simulink model "LIM"  (R2022b)
settings: Solver=VariableStepAuto  StartTime=0.0  StopTime=2  RelTol=1e-3
model workspace (MAT data in the model file):
  F = Simulink.Parameter
  F.DataType = 'auto'
  F.Complexity = 'real'
  F.Dimensions = [0 0]
values from neighbouring files (symbols this model uses):
  B = 0.93    [proj.m]
  D = 2.150    (= 2.15)    [proj.m]
  Llr = 0.0323    [proj.m]
  Lls = 0.0788    [proj.m]
  Lm = 0.0420    (= 0.042)    [proj.m]
  M = 16.1    [proj.m]
  P = 2    [proj.m]
  Rr = 10.166    [proj.m]
  Rs = 1.6875    [proj.m]
  Vo = 220    [proj.m]
  Ws = 314.5    [proj.m]
libraries: spspowerguiLib x1
settings Model: Creator=Hassan Alam  LastModifiedBy=DELL
settings SolverCC: AlgebraicLoopSolver=TrustRegion
settings DebuggingCC: UnconnectedInputMsg=warning  UnconnectedOutputMsg=warning  UnconnectedLineMsg=warning  SFMachineParentedDataDiag=warning  ArithmeticOperatorsInVariantConditions=warning
settings ModelReferenceCC: EnableRefExpFcnMdlSchedulingChecks=on
settings SFSimCC: CustomCodeUndefinedFunction=UseInterfaceOnly
settings RTWCC: DLArmComputeVersion=19.05

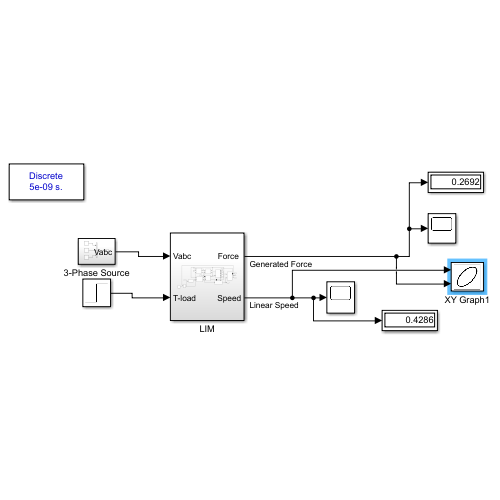
[thumbnail: Simulink's stored preview of the top-level diagram]
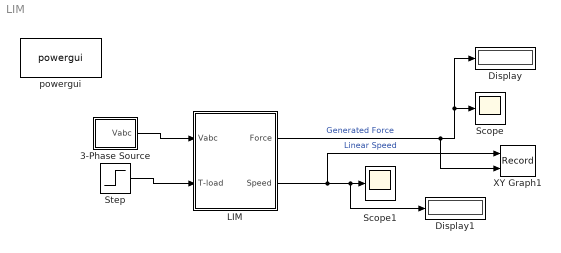
== system LIM ==
  3-Phase Source : Subsystem
  Display : Display
  Display1 : Display
  LIM : Subsystem
  Scope : Scope
  Scope1 : Scope
  Step : Step  Time=2  After=2  SampleTime=0
  XY Graph1 : Record  FileSettingsInternal="{\"entries\":[{\"content\":{\"excelSettings\":{\"content\":{},\"type\":\"Streamout.ExcelSettings\"}},\"type\":\"Streamout.FileSettingStorage\",\"uuid\":\"f2251dd7-1574-4eda-90b9-688bc1165eb5\"}],\"packageUris\":[\"http://schema.mathworks.com/mf0/streamout_blocks/R2020a\"],\"version\":\"1.0\"}"  Layout=[1 1]  SignalsInternal="{\"entries\":[{\"content\":{\"signals\":[{\"content\":{\"blockPath\":[\"Linear_IM/XY Graph1\"],\"channel\":[],\"dimensions\":[1],\"domain\":\"Linear_IM/XY Graph1\",\"lineColor\":\"#a2142f\",\"plots\":[1],\"port\":1,\"sid\":[],\"signalID\":8,\"signalName\":\"Linear Speed\"},\"type\":\"RecordBlkView.Signal\",\"uuid\":\"07500a95-6970-4b1d-b2d0-133414292f8e\"},{\"content\":{\"blockPath\":[\"Linear_IM/XY Graph1\"],\"channel\":[],\"dimensions\":[1],\"domain\":\"Linear_IM/XY Graph1\",\"lineColor\":\"#139fff\",\"plots\":[1],\"port\":2,\"sid\":[],\"signalID\":11,\"signalName\":\"Generated Force\"},\"type\":\"RecordBlkView.Signal\",\"uuid\":\"d5d04c6d-1390-4e30-b79d-0de345d9fcfb\"}]},\"type\":\"RecordBlkView.InputSignals\",\"uuid\":\"6577f966-2e08-44dc-8997-1caec95d4b14\"}],\"packageUris\":[\"http://schema.mathworks.com/mf0/streamout_blocks/R2020a\"],\"version\":\"1.0\"}"  VisualizationBindings="{\"xyplotplugin\":{\"info\":[{\"series\":[{\"bindingParametersList\":[{\"parameter\":\"X-Axis\",\"signalID\":8,\"signalName\":\"Linear Speed\"},{\"parameter\":\"Y-Axis\",\"signalID\":11,\"signalName\":\"Generated Force\"}],\"seriesID\":8522}],\"subplotID\":1}]}}"  CompatibilityTag=XY
  powergui : spspowerguiLib/powergui  Priority=1  SimulationMode=Discrete  SampleTime=50e-10  frequency=60  Iterations=50  frequencyindice=60  Pbase=100e6  ErrMax=1e-4  UnitsV=kV  UnitsW=MW  buscounter=0  FunctionMessages=off  echomessages=off  EnableUseOfTLC=off  CurrentSourceSwitches=off  DisableSnubberDevices=off  DisableRonSwitches=off  DisableVfSwitches=off  DisplayEquations=off  AutomaticDiscreteSolvers=off  SolverType=Tustin/Backward Euler (TBE)  Interpol=off  ExternalGateDelay=off  methode=off  Ts=100  x0status=blocks  SPID=on  SwTol=0  HookPort=off  NonlinearTolerance=1e-4  nMaxIteration=100  ContinueOnMaxIteration=off  RestoreLinks=warning  ResistiveCurrentMeasurement=off  Frange=[0:2:500]  Ylog=off  Xlog=on  ShowGrid=off  save=off  variable=ZData  structure=0  ZoomFFT=off  StartTime=0.0  cycles=1  DisplayStyle=1  fundamental=60  FreqAxis=off  MaxFrequency=1000  frequencyindicesteady=1  RmsSteady=1  display=off
  wires:
  Step/1 -> LIM/2(T-load)
  LIM/1("Force ") -> XY Graph1/2, Display/1, Scope/1  "Generated Force"
  LIM/2(" Speed") -> XY Graph1/1, Scope1/1, Display1/1  "Linear Speed"
  3-Phase Source/1(Vabc) -> LIM/1(Vabc)

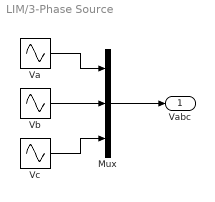
== system LIM/3-Phase Source ==
  Mux : Mux  Inputs=3
  Va : Sin  Amplitude=Vo  Frequency=Ws  SampleTime=0
  Vb : Sin  Amplitude=Vo  Frequency=Ws  Phase=-2*pi/3  SampleTime=0
  Vc : Sin  Amplitude=Vo  Frequency=Ws  Phase=2*pi/3  SampleTime=0
  Vabc : Outport
  wires:
  Mux/1 -> Vabc/1
  Vb/1 -> Mux/2
  Va/1 -> Mux/1
  Vc/1 -> Mux/3

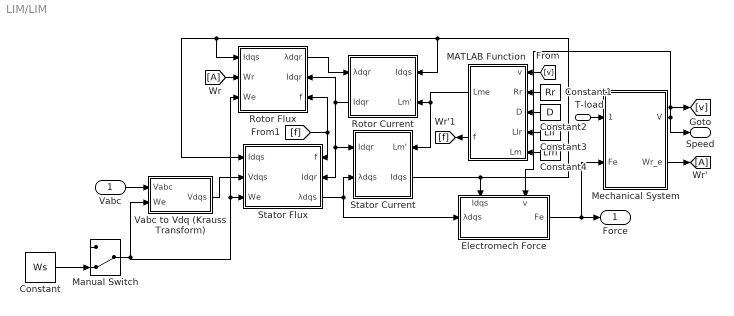
== system LIM/LIM ==
  Vabc : Inport
  T-load : Inport  Port=2
  Constant : Constant  Value=Ws
  Constant1 : Constant  Value=Rr
  Constant2 : Constant  Value=D
  Constant3 : Constant  Value=Llr
  Constant4 : Constant  Value=Lm
  Electromech Force : Subsystem
      settings: PortSchema="{\"entries\":[{\"content\":{\"sides\":[{\"content\":{\"connectorIds\":[\"In1\"]},\"type\":\"ConnectorPlacement.EquallySpacedRectSide\",\"uuid\":\"a4b29cca-9cb0-4324-9244-2049ffc93668\"},{\"content\":{\"connectorIds\":[\"Out1\"],\"side\":\"RIGHT\"},\"type\":\"ConnectorPlacement.EquallySpacedRectSide\",\"uuid\":\"b20ff3ac-d40e-4f59-bb91-f6f2c0c6ca63\"},{\"content\":{\"connectorIds\":[\"In2\",\"In3\"],\"side\":\"TOP\"},\"type\":\"ConnectorPlacement.EquallySpacedRectSide\",\"uuid\":\"55342d43-b8f9-4aa9-846c-26670e92f4ca\"},{\"content\":{\"connectorIds\":[],\"side\":\"HIDDEN\"},\"type\":\"ConnectorPlacement.EquallySpacedRectSide\",\"uuid\":\"5fed22a0-a45a-430c-a997-0be85a9315bb\"}]},\"type\":\"ConnectorPlacement.EquallySpacedConnector\",\"uuid\":\"78d5652d-2b6b-4c50-974b-d09ad892483f\"}],\"packageUris\":[\"http://schema.mathworks.com/mf0/Connector/R2020b\"],\"version\":\"1.0\"}"
  MATLAB Function : MATLAB Function  TreatAsAtomicUnit=on
  Manual Switch : ManualSwitch  CurrentSetting=0
  Mechanical System : Subsystem
  Rotor Current : Subsystem
      settings: PortSchema="{\"entries\":[{\"content\":{\"sides\":[{\"content\":{\"connectorIds\":[\"In1\",\"Out1\"]},\"type\":\"ConnectorPlacement.EquallySpacedRectSide\",\"uuid\":\"b9a9f404-9b3b-4182-a50e-1bf7cef191e8\"},{\"content\":{\"connectorIds\":[\"In2\",\"In3\"],\"side\":\"RIGHT\"},\"type\":\"ConnectorPlacement.EquallySpacedRectSide\",\"uuid\":\"68159d79-7975-4fd0-98a3-7e35432781a2\"},{\"content\":{\"connectorIds\":[],\"side\":\"TOP\"},\"type\":\"ConnectorPlacement.EquallySpacedRectSide\",\"uuid\":\"0c4dbb5d-b4d4-4876-b829-49090bd6eeb8\"},{\"content\":{\"connectorIds\":[],\"side\":\"BOTTOM\"},\"type\":\"ConnectorPlacement.EquallySpacedRectSide\",\"uuid\":\"e42509db-2e5f-42f8-9a91-9046ba95e836\"},{\"content\":{\"connectorIds\":[],\"side\":\"HIDDEN\"},\"type\":\"ConnectorPlacement.EquallySpacedRectSide\",\"uuid\":\"f2a65973-682a-4dd6-b429-3fa72198cae4\"}]},\"type\":\"ConnectorPlacement.EquallySpacedConnector\",\"uuid\":\"744eb17f-cf6a-4151-90db-78263b57d619\"}],\"packageUris\":[\"http://schema.mathworks.com/mf0/Connector/R2020b\"],\"version\":\"1.0\"}"
  Rotor Flux : Subsystem
      settings: PortSchema="{\"entries\":[{\"content\":{\"sides\":[{\"content\":{\"connectorIds\":[\"In1\",\"In2\",\"In3\"]},\"type\":\"ConnectorPlacement.EquallySpacedRectSide\",\"uuid\":\"b9a9f404-9b3b-4182-a50e-1bf7cef191e8\"},{\"content\":{\"connectorIds\":[\"Out1\",\"In4\",\"In5\"],\"side\":\"RIGHT\"},\"type\":\"ConnectorPlacement.EquallySpacedRectSide\",\"uuid\":\"68159d79-7975-4fd0-98a3-7e35432781a2\"},{\"content\":{\"connectorIds\":[],\"side\":\"TOP\"},\"type\":\"ConnectorPlacement.EquallySpacedRectSide\",\"uuid\":\"0c4dbb5d-b4d4-4876-b829-49090bd6eeb8\"},{\"content\":{\"connectorIds\":[],\"side\":\"HIDDEN\"},\"type\":\"ConnectorPlacement.EquallySpacedRectSide\",\"uuid\":\"f2a65973-682a-4dd6-b429-3fa72198cae4\"}]},\"type\":\"ConnectorPlacement.EquallySpacedConnector\",\"uuid\":\"744eb17f-cf6a-4151-90db-78263b57d619\"}],\"packageUris\":[\"http://schema.mathworks.com/mf0/Connector/R2020b\"],\"version\":\"1.0\"}"
  Stator Current : Subsystem
      settings: PortSchema="{\"entries\":[{\"content\":{\"sides\":[{\"content\":{\"connectorIds\":[\"In1\",\"In2\"]},\"type\":\"ConnectorPlacement.EquallySpacedRectSide\",\"uuid\":\"c6a8d684-b7d2-4173-9e8a-0a77b360fa3b\"},{\"content\":{\"connectorIds\":[\"In3\",\"Out1\"],\"side\":\"RIGHT\"},\"type\":\"ConnectorPlacement.EquallySpacedRectSide\",\"uuid\":\"6b547613-238c-47a7-9a25-113e0bcf67e8\"},{\"content\":{\"connectorIds\":[],\"side\":\"TOP\"},\"type\":\"ConnectorPlacement.EquallySpacedRectSide\",\"uuid\":\"9eb731ca-d22d-4bff-90d4-9f452150afc4\"},{\"content\":{\"connectorIds\":[],\"side\":\"HIDDEN\"},\"type\":\"ConnectorPlacement.EquallySpacedRectSide\",\"uuid\":\"3386087c-4273-46bf-b0bc-9959c9fde15b\"}]},\"type\":\"ConnectorPlacement.EquallySpacedConnector\",\"uuid\":\"3fded039-aa6e-4722-8a98-01f4cd5eabc0\"}],\"packageUris\":[\"http://schema.mathworks.com/mf0/Connector/R2020b\"],\"version\":\"1.0\"}"
  Stator Flux : Subsystem
      settings: PortSchema="{\"entries\":[{\"content\":{\"sides\":[{\"content\":{\"connectorIds\":[\"In1\",\"In2\",\"In3\"]},\"type\":\"ConnectorPlacement.EquallySpacedRectSide\",\"uuid\":\"a4b29cca-9cb0-4324-9244-2049ffc93668\"},{\"content\":{\"connectorIds\":[\"In4\",\"In5\",\"Out1\"],\"side\":\"RIGHT\"},\"type\":\"ConnectorPlacement.EquallySpacedRectSide\",\"uuid\":\"b20ff3ac-d40e-4f59-bb91-f6f2c0c6ca63\"},{\"content\":{\"connectorIds\":[],\"side\":\"TOP\"},\"type\":\"ConnectorPlacement.EquallySpacedRectSide\",\"uuid\":\"55342d43-b8f9-4aa9-846c-26670e92f4ca\"},{\"content\":{\"connectorIds\":[],\"side\":\"HIDDEN\"},\"type\":\"ConnectorPlacement.EquallySpacedRectSide\",\"uuid\":\"5fed22a0-a45a-430c-a997-0be85a9315bb\"}]},\"type\":\"ConnectorPlacement.EquallySpacedConnector\",\"uuid\":\"78d5652d-2b6b-4c50-974b-d09ad892483f\"}],\"packageUris\":[\"http://schema.mathworks.com/mf0/Connector/R2020b\"],\"version\":\"1.0\"}"
  Vabc to Vdq (Krauss Transform) : Subsystem
  Wr : From
  Wr' : Goto
  "Force " : Outport
  " Speed" : Outport  Port=2
  wires:
  Electromech Force/1(Fe) -> Mechanical System/2(Fe), "Force "/1
  T-load/1 -> Mechanical System/1(F-load)
  Mechanical System/1(V) -> Electromech Force/3(v), [v], " Speed"/1
  Stator Flux/1(λdqs) -> Stator Current/2(λdqs), Electromech Force/1(λdqs)
  Stator Current/1(Idqs) -> Rotor Flux/1(Idqs), Stator Flux/1(Idqs), Rotor Current/2(Idqs), Electromech Force/2(Idqs)
  Rotor Flux/1(λdqr) -> Rotor Current/1(λdqr)
  Rotor Current/1(Idqr) -> Rotor Flux/4(Idqr), Stator Flux/5(Idqr), Stator Current/1(Idqr)
  Wr/1 -> Rotor Flux/2(Wr)
  Vabc/1 -> Vabc to Vdq (Krauss Transform)/1(Vabc)
  Vabc to Vdq (Krauss Transform)/1(Vdqs) -> Stator Flux/2(Vdqs)
  MATLAB Function/1(Lme) -> Stator Current/3(Lm'), Rotor Current/3(Lm')
  [v] -> MATLAB Function/1(v)
  Constant1/1 -> MATLAB Function/2(Rr)
  Constant2/1 -> MATLAB Function/3(D)
  Constant3/1 -> MATLAB Function/4(Llr)
  Constant4/1 -> MATLAB Function/5(Lm)
  MATLAB Function/2(f) -> [f]
  [f] -> Rotor Flux/5(f), Stator Flux/4(f)
  Mechanical System/2(Wr_e) -> Wr'/1
  Manual Switch/1 -> Rotor Flux/3(We), Stator Flux/3(We), Vabc to Vdq (Krauss Transform)/2(We)
  Constant/1 -> Manual Switch/2

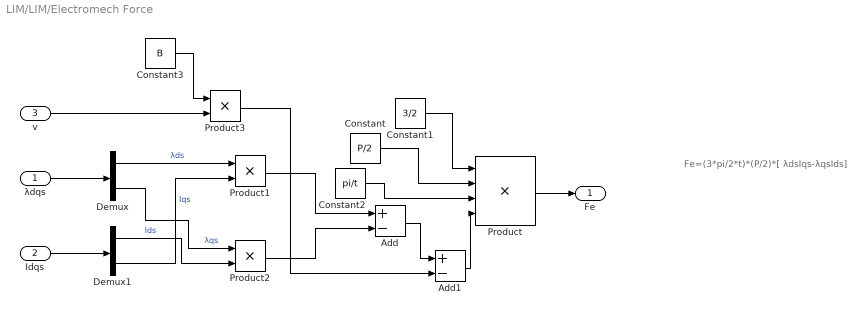
== system LIM/LIM/Electromech Force ==
  note: Fe=(3*pi/2*t)*(P/2)*[ λdsIqs-λqsIds]
  λdqs : Inport
  Idqs : Inport  Port=2
  v : Inport  Port=3
  Add : Sum  Inputs=+-
  Add1 : Sum  Inputs=+-
  Constant : Constant  Value=P/2
  Constant1 : Constant  Value=3/2
  Constant2 : Constant  Value=pi/t
  Constant3 : Constant  Value=B
  Demux : Demux  Outputs=2
  Demux1 : Demux  Outputs=2
  Product : Product  Inputs=4
  Product1 : Product
  Product2 : Product
  Product3 : Product
  Fe : Outport
  wires:
  Product/1 -> Fe/1
  Constant1/1 -> Product/1
  λdqs/1 -> Demux/1
  Idqs/1 -> Demux1/1
  Demux/1 -> Product1/1  "λds"
  Demux1/2 -> Product1/2  "Iqs"
  Demux/2 -> Product2/1  "λqs"
  Demux1/1 -> Product2/2  "Ids"
  Product1/1 -> Add/1
  Product2/1 -> Add/2
  Constant2/1 -> Product/3
  Constant/1 -> Product/2
  v/1 -> Product3/2
  Add/1 -> Add1/1
  Add1/1 -> Product/4
  Product3/1 -> Add1/2
  Constant3/1 -> Product3/1

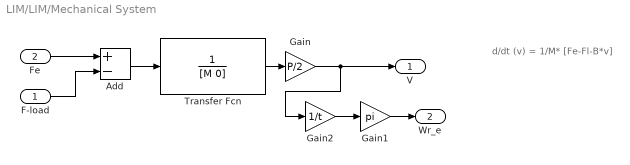
== system LIM/LIM/Mechanical System ==
  note: d/dt (v) = 1/M* [Fe-Fl-B*v]
  F-load : Inport
  Fe : Inport  Port=2
  Add : Sum  Inputs=+-
  Gain : Gain  Gain=P/2
  Gain1 : Gain  Gain=pi
  Gain2 : Gain  Gain=1/t
  Transfer Fcn : TransferFcn  Denominator=[M 0]
  V : Outport
  Wr_e : Outport  Port=2
  wires:
  Fe/1 -> Add/1
  F-load/1 -> Add/2
  Add/1 -> Transfer Fcn/1
  Gain2/1 -> Gain1/1
  Gain1/1 -> Wr_e/1
  Gain/1 -> Gain2/1, V/1
  Transfer Fcn/1 -> Gain/1

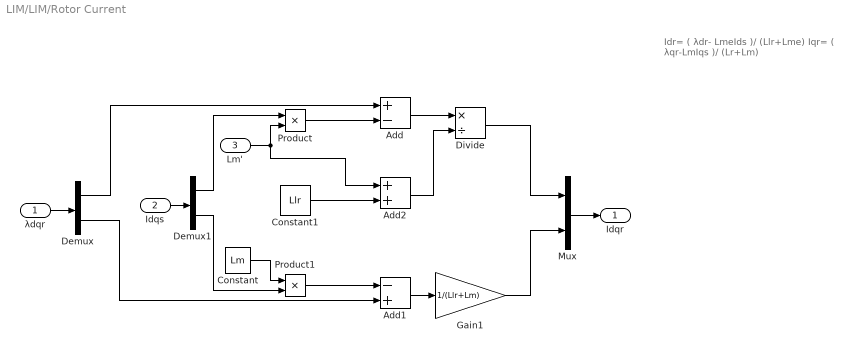
== system LIM/LIM/Rotor Current ==
  note: Idr= ( λdr- LmeIds )/ (Llr+Lme)
      |
      | Iqr= ( λqr-LmIqs )/ (Lr+Lm)
  λdqr : Inport
  Idqs : Inport  Port=2
  Lm' : Inport  Port=3
  Add : Sum  Inputs=+-
  Add1 : Sum  Inputs=-+
  Add2 : Sum
  Constant : Constant  Value=Lm  VectorParams1D=off
  Constant1 : Constant  Value=Llr
  Demux : Demux  Outputs=2
  Demux1 : Demux  Outputs=2
  Divide : Product  Inputs=*/
  Gain1 : Gain  Gain=1/(Llr+Lm)
  Mux : Mux  Inputs=2
  Product : Product
  Product1 : Product
  Idqr : Outport
  wires:
  Mux/1 -> Idqr/1
  λdqr/1 -> Demux/1
  Idqs/1 -> Demux1/1
  Demux1/1 -> Product/1
  Demux1/2 -> Product1/2
  Demux/1 -> Add/1
  Demux/2 -> Add1/2
  Product/1 -> Add/2
  Product1/1 -> Add1/1
  Add/1 -> Divide/1
  Add1/1 -> Gain1/1
  Gain1/1 -> Mux/2
  Divide/1 -> Mux/1
  Constant/1 -> Product1/1
  Constant1/1 -> Add2/2
  Lm'/1 -> Add2/1, Product/2
  Add2/1 -> Divide/2

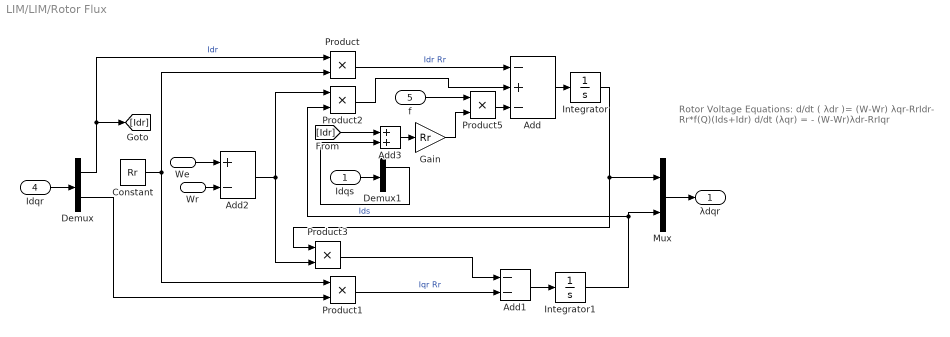
== system LIM/LIM/Rotor Flux ==
  note: Rotor Voltage Equations:
      | d/dt ( λdr )= (W-Wr) λqr-RrIdr- Rr*f(Q)(Ids+Idr)
      | d/dt (λqr) = - (W-Wr)λdr-RrIqr
  Idqs : Inport
  Wr : Inport  Port=2
  We : Inport  Port=3
  Idqr : Inport  Port=4
  f : Inport  Port=5
  Add : Sum  Inputs=-+-
  Add1 : Sum  Inputs=--
  Add2 : Sum  Inputs=+-
  Add3 : Sum
  Constant : Constant  Value=Rr
  Demux : Demux  Outputs=2
  Demux1 : Demux  Outputs=2
  Gain : Gain  Gain=Rr
  Integrator : Integrator
  Integrator1 : Integrator
  Mux : Mux  Inputs=2
  Product{,1..3,5} (5 alike) : Product
  λdqr : Outport
  wires:
  Mux/1 -> λdqr/1
  Idqr/1 -> Demux/1
  Demux/1 -> [Idr], Product/1  "Idr"
  Demux/2 -> Product1/2
  Constant/1 -> Product1/1, Product/2
  Product/1 -> Add/1  "Idr Rr"
  Product1/1 -> Add1/2  "Iqr Rr"
  Add/1 -> Integrator/1
  Add1/1 -> Integrator1/1
  Integrator1/1 -> Mux/2, Product2/2
  Integrator/1 -> Product3/1, Mux/1
  We/1 -> Add2/1
  Wr/1 -> Add2/2
  Add2/1 -> Product3/2, Product2/1
  Product2/1 -> Add/2
  Product3/1 -> Add1/1
  Demux1/1 -> Add3/2  "Ids"
  Product5/1 -> Add/3
  Add3/1 -> Gain/1
  Gain/1 -> Product5/2
  f/1 -> Product5/1
  Idqs/1 -> Demux1/1
  [Idr] -> Add3/1

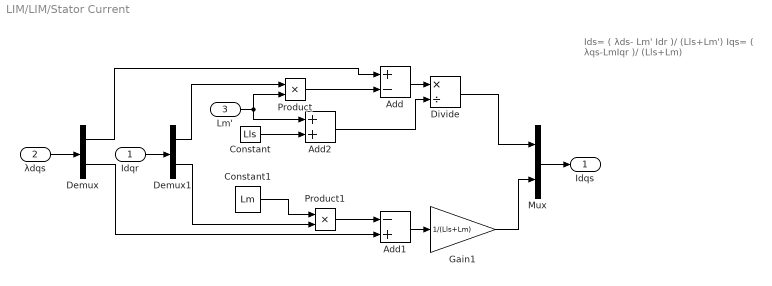
== system LIM/LIM/Stator Current ==
  note: Ids= ( λds- Lm' Idr )/ (Lls+Lm')
      |
      | Iqs= ( λqs-LmIqr )/ (Lls+Lm)
  Idqr : Inport
  λdqs : Inport  Port=2
  Lm' : Inport  Port=3
  Add : Sum  Inputs=+-
  Add1 : Sum  Inputs=-+
  Add2 : Sum
  Constant : Constant  Value=Lls
  Constant1 : Constant  Value=Lm  VectorParams1D=off
  Demux : Demux  Outputs=2
  Demux1 : Demux  Outputs=2
  Divide : Product  Inputs=*/
  Gain1 : Gain  Gain=1/(Lls+Lm)
  Mux : Mux  Inputs=2
  Product : Product
  Product1 : Product
  Idqs : Outport
  wires:
  Demux/2 -> Add1/2
  Demux1/1 -> Product/1
  Product/1 -> Add/2
  Product1/1 -> Add1/1
  λdqs/1 -> Demux/1
  Add1/1 -> Gain1/1
  Mux/1 -> Idqs/1
  Idqr/1 -> Demux1/1
  Demux/1 -> Add/1
  Demux1/2 -> Product1/2
  Add/1 -> Divide/1
  Divide/1 -> Mux/1
  Gain1/1 -> Mux/2
  Constant1/1 -> Product1/1
  Lm'/1 -> Add2/1, Product/2
  Constant/1 -> Add2/2
  Add2/1 -> Divide/2

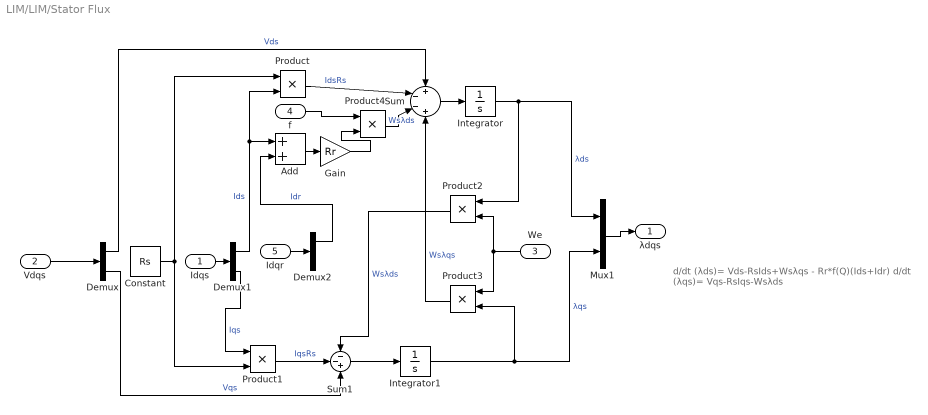
== system LIM/LIM/Stator Flux ==
  note: d/dt (λds)= Vds-RsIds+Wsλqs - Rr*f(Q)(Ids+Idr)
      |
      | d/dt (λqs)= Vqs-RsIqs-Wsλds
  Idqs : Inport
  Vdqs : Inport  Port=2
  We : Inport  Port=3
  f : Inport  Port=4
  Idqr : Inport  Port=5
  Add : Sum
  Constant : Constant  Value=Rs
  Demux : Demux  Outputs=2
  Demux1 : Demux  Outputs=2
  Demux2 : Demux  Outputs=2
  Gain : Gain  Gain=Rr
  Integrator : Integrator
  Integrator1 : Integrator
  Mux1 : Mux  Inputs=2
  Product{,1..4} (5 alike) : Product
  Sum : Sum  Inputs=+--+
  Sum1 : Sum  Inputs=--+
  λdqs : Outport
  wires:
  Integrator1/1 -> Product3/2, Mux1/2  "λqs"
  Integrator/1 -> Product2/1, Mux1/1  "λds"
  Vdqs/1 -> Demux/1
  Idqs/1 -> Demux1/1
  Demux/1 -> Sum/1  "Vds"
  Sum/1 -> Integrator/1
  Constant/1 -> Product1/2, Product/1
  Demux1/1 -> Product/2, Add/1  "Ids"
  Product/1 -> Sum/2  "IdsRs"
  Sum1/1 -> Integrator1/1
  Demux/2 -> Sum1/3  "Vqs"
  Demux1/2 -> Product1/1  "Iqs"
  Product1/1 -> Sum1/2  "IqsRs"
  We/1 -> Product3/1, Product2/2
  Product3/1 -> Sum/4  "Wsλqs"
  Product2/1 -> Sum1/1  "Wsλds"
  Mux1/1 -> λdqs/1
  Idqr/1 -> Demux2/1
  Demux2/1 -> Add/2  "Idr"
  Add/1 -> Gain/1
  Gain/1 -> Product4/2
  Product4/1 -> Sum/3  "Wsλds"
  f/1 -> Product4/1

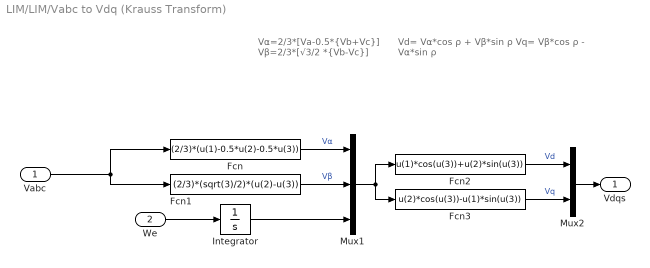
== system LIM/LIM/Vabc to Vdq (Krauss Transform) ==
  note: Vα=2/3*[Va-0.5*{Vb+Vc}]
      |
      | Vβ=2/3*[√3/2 *{Vb-Vc}]
  note: Vd= Vα*cos ρ + Vβ*sin ρ
      |
      | Vq= Vβ*cos ρ - Vα*sin ρ
  Vabc : Inport
  We : Inport  Port=2
  Fcn : Fcn  Expr=(2/3)*(u(1)-0.5*u(2)-0.5*u(3))
  Fcn1 : Fcn  Expr=(2/3)*(sqrt(3)/2)*(u(2)-u(3))
  Fcn2 : Fcn  Expr=u(1)*cos(u(3))+u(2)*sin(u(3))
  Fcn3 : Fcn  Expr=u(2)*cos(u(3))-u(1)*sin(u(3))
  Integrator : Integrator
  Mux1 : Mux  Inputs=3
  Mux2 : Mux  Inputs=2
  Vdqs : Outport
  wires:
  Fcn/1 -> Mux1/1  "Vα"
  Fcn1/1 -> Mux1/2  "Vβ"
  Vabc/1 -> Fcn/1, Fcn1/1
  Mux2/1 -> Vdqs/1
  We/1 -> Integrator/1
  Integrator/1 -> Mux1/3
  Fcn2/1 -> Mux2/1  "Vd"
  Mux1/1 -> Fcn3/1, Fcn2/1
  Fcn3/1 -> Mux2/2  "Vq"

== matlab function LIM/MATLAB Function ==
  data: v input; Lme output; Rr input; D input; Llr input; Lm input; f output
function [Lme,f]= fcn(v, Rr,D,Llr,Lm)
Q=abs((D*Rr)/(Llr*v)); % q is not charge but a factor related to not only the primary
%length but also the machine velocity
f=(1-(exp(-Q)))/Q; % this is the equation for end effect
Lme = Lm*(1-f)  % reduction in magnetization current due to end effect
